simulink model "Final_Model_obs"  (R2024a)
settings: Solver=VariableStepAuto  StartTime=0.0  StopTime=10.0  RelTol=1e-3
values from neighbouring files (symbols this model uses):
  A = [0 1 0 ... (first row only)    [K_mat.m]    (also in init.m)
  B = [0 ... (first row only)    [K_mat.m]    (also in init.m)
  C = [1 0 0 ... (first row only)    [init.m]
  G = 5    [K_mat.m]    (also in init.m)
  H = 1    [K_mat.m]    (also in init.m)
  K = -V/Z    [solveKMatrix_class.m]
  K0 = K0_T'    [observe.m]
  L = 20    [K_mat.m]    (also in init.m)
  M = 100    [K_mat.m]    (also in init.m)
  R = 3    [K_mat.m]    (also in control.m = 1; init.m)
  x_ref = [0.01, 0, 0.002]    [control.m]
settings Model: Creator=casager  LastModifiedBy=casager

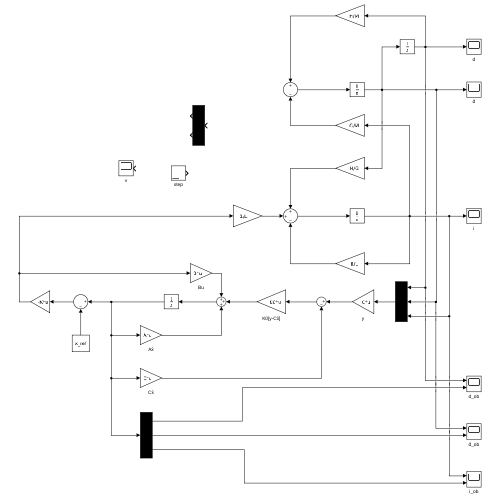
[thumbnail: Simulink's stored preview of the top-level diagram]
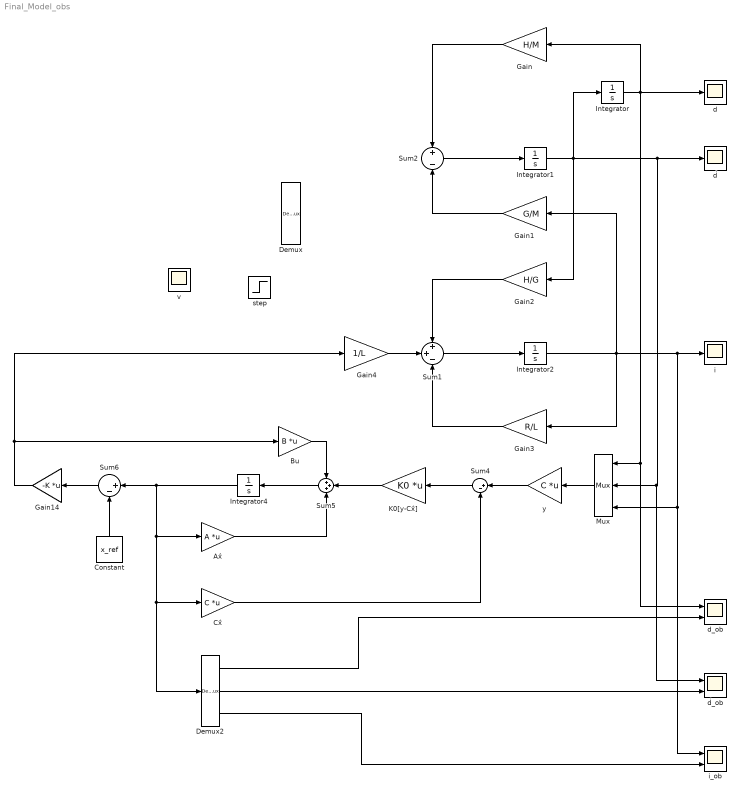
== system Final_Model_obs ==
  Ax̂ : Gain  Gain=A  Multiplication=Matrix(K*u)
  Bu : Gain  Gain=B  Multiplication=Matrix(K*u)
  Constant : Constant  Value=x_ref
  Cx̂ : Gain  Gain=C  Multiplication=Matrix(K*u)
  Demux : Demux  Outputs=2
  Demux2 : Demux  Outputs=3
  Gain : Gain  Gain=H/M
  Gain1 : Gain  Gain=G/M
  Gain14 : Gain  Gain=-K  Multiplication=Matrix(K*u)
  Gain2 : Gain  Gain=H/G
  Gain3 : Gain  Gain=R/L
  Gain4 : Gain  Gain=1/L
  Integrator : Integrator  InitialCondition=0.015
  Integrator1 : Integrator
  Integrator2 : Integrator
  Integrator4 : Integrator
  K0[y-Cx̂] : Gain  Gain=K0  Multiplication=Matrix(K*u)
  Mux : Mux  Inputs=3
  Sum1 : Sum  Inputs=++-
  Sum2 : Sum  Inputs=+-
  Sum4 : Sum  Inputs=|+-
  Sum5 : Sum  Inputs=+++
  Sum6 : Sum  Inputs=|+-
  d : Scope
  d_ob : Scope  NumInputPorts=2
  i : Scope
  i_ob : Scope  NumInputPorts=2
  step : Step  After=100  SampleTime=0
  v : Scope
  y : Gain  Gain=C  Multiplication=Matrix(K*u)
  ḋ : Scope
  ḋ_ob : Scope  NumInputPorts=2
  wires:
  Integrator/1 -> d_ob/1, Mux/1, Gain/1, d/1
  Sum1/1 -> Integrator2/1
  Gain/1 -> Sum2/1
  Gain1/1 -> Sum2/2
  Integrator1/1 -> Integrator/1, Gain2/1, ḋ_ob/1, Mux/2, ḋ/1
  Gain2/1 -> Sum1/1
  Sum2/1 -> Integrator1/1
  Gain3/1 -> Sum1/3
  Gain4/1 -> Sum1/2
  Integrator2/1 -> Gain1/1, i_ob/1, Mux/3, i/1, Gain3/1
  K0[y-Cx̂]/1 -> Sum5/2
  Sum5/1 -> Integrator4/1
  Ax̂/1 -> Sum5/3
  Sum4/1 -> K0[y-Cx̂]/1
  Cx̂/1 -> Sum4/2
  Gain14/1 -> Gain4/1, Bu/1
  Integrator4/1 -> Sum6/1, Ax̂/1, Demux2/1, Cx̂/1
  Bu/1 -> Sum5/1
  Mux/1 -> y/1
  Sum6/1 -> Gain14/1
  Constant/1 -> Sum6/2
  y/1 -> Sum4/1
  Demux2/2 -> ḋ_ob/2
  Demux2/1 -> d_ob/2
  Demux2/3 -> i_ob/2
